simulink library "library"  (R2023a)
settings: Solver=VariableStepAuto  StartTime=0.0  StopTime=10.0  RelTol=1e-3
settings Model: Creator=miria  LastModifiedBy=miria

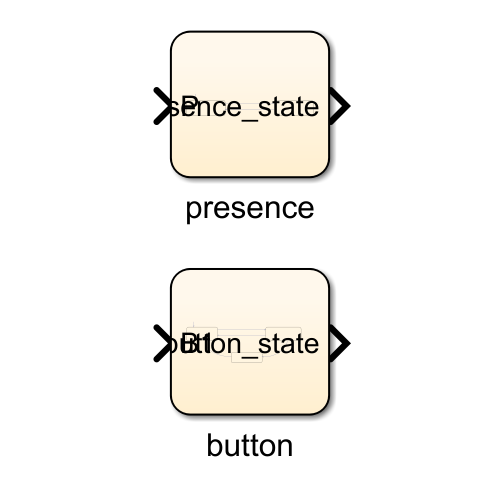
[thumbnail: Simulink's stored preview of the top-level diagram]
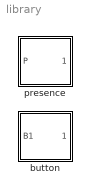
== system library ==
  button : Stateflow chart  TreatAsAtomicUnit=on
  presence : Stateflow chart  TreatAsAtomicUnit=on

== stateflow chart library/presence ==
  state wait
    en: presence_state = ~PRESENCE;
  state pressed
    en: presence_state = ~PRESENCE;
    on after(0.5, sec):
    presence_state = PRESENCE;
  (default) -> wait
  wait -> pressed : [P == PRESENCE]
  pressed -> wait : [P ~= PRESENCE]
  data: P input boolean size=1; presence_state output boolean size=1; PRESENCE constant boolean =0

== stateflow chart library/button ==
  state wait
    en: button_state = RELEASED;
  state pressed
    en: button_state = RELEASED;
    on after(BUTTONDURATION, sec):
    button_state = PRESSED;
  state longpressed
    en: button_state = RELEASED;
  (default) -> wait
  wait -> pressed : [B1 == PRESSED]
  pressed -> wait [order 2] : [B1 == RELEASED]
  longpressed -> wait : [B1 == RELEASED]
  pressed -> longpressed [order 1] : [button_state == PRESSED & B1 == PRESSED]
  data: B1 input; BUTTONDURATION parameter double; PRESSED constant boolean =0; RELEASED constant boolean =1; button_state output boolean size=1
